simulink model "udp_conn"  (R2016b)
settings: Solver=FixedStepDiscrete  StartTime=0.0  StopTime=5  RelTol=1e-3  EnableMultiTasking=on
undefined symbols (not defined in the file): sldrtexcb_modeswitch, Standard_Devices, UDP_Protocol
libraries: sldrtlib x4, xpcseriallib x1
Description:
  | Packet Input/Output
  | 
  | The example model "sldrtex_packetio" shows how to transfer data through UDP
  | communication protocol using binary encoding. The model sends data
  | within one computer, from one UDP port to another. You can modify the
  | model to communicate between two computers by splitting this model
  | into its send and receive parts and running the models on two computers.
  | The yellow blocks are used to send the data, the blue blocks
  | are used to receive the data. Then, please enter the IP addresses of the two
  | computers into the appropriate fields in the Board Setup dialog.
  | 
  | How to run this model in Normal Mode:
  | 
  | 1) Double-click the orange button to switch to Normal Mode if needed.
  | 2) Start the real-time execution using Simulation->Run.
  | 
  | How to run this model in External Mode:
  | 
  | 1) Double-click the orange button to switch to External Mode if needed.
  | 2) Start the real-time execution using Simulation->Run. The model will automatically
  |    build, connect to Simulink in External Mode and start.
settings Model: SimulationMode=external  ExtModeTrigDuration=1001  Creator=The MathWorks, Inc.  LastModifiedBy=gylaszlo
settings DataIOCC: LimitDataPoints=on  SaveFormat=Array
settings OptimizationCC: ExpressionDepthLimit=2147483647  InitFltsAndDblsToZero=on  EfficientMapNaN2IntZero=off  LifeSpan=inf
settings DebuggingCC: UnderspecifiedInitializationDetection=Classic  MergeDetectMultiDrivingBlocksExec=none  SolverPrmCheckMsg=warning  FcnCallInpInsideContextMsg=warning  AllowSymbolicDim=off  StateNameClashWarn=warning  SFUnexpectedBacktrackingDiag=warning  SFNoUnconditionalDefaultTransitionDiag=warning  SFExecutionAtInitializationDiag=none
settings HardwareCC: TargetBitPerLong=64  TargetBitPerPointer=64  TargetBitPerSizeT=64  TargetBitPerPtrDiffT=64  TargetIntDivRoundTo=Zero  TargetEndianess=LittleEndian  TargetWordSize=64  TargetHWDeviceType=Intel->x86-64
settings ModelReferenceCC: PropagateSignalLabelsOutOfModel=off
settings RTWCC: SystemTargetFile=sldrt.tlc  TemplateMakefile=sldrt.tmf  Description=Simulink Desktop Real-Time  RTWCompilerOptimization=on
settings CodeAppCC: MaxIdLength=95
settings SimulinkDesktopRealTimeCC: TargetPreCompLibLocation=C:\Program Files\MATLAB\R2016b\toolbox\sldrt\lib\win64  TargetLangStandard=C89/C90 (ANSI)  GeneratePreprocessorConditionals=Disable all  SupportVariableSizeSignals=off
settings ConfigComp: CovMetricSettings=dw  CovHtmlReporting=on  CovSaveCumulativeToWorkspaceVar=on  CovSaveSingleToWorkspaceVar=on  CovShowResultsExplorer=off  CovExternalEMLEnable=off  CovSFcnEnable=off

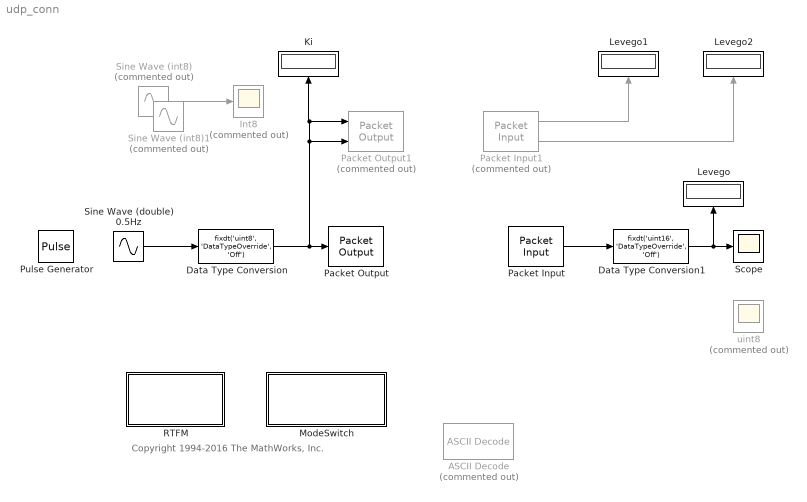
== system udp_conn ==
  note: Copyright 1994-2016 The MathWorks, Inc.
  "ASCII Decode " : xpcseriallib/ASCII Decode   Commented=on  format=%d\r  nvars=1  vartypes={ }
  Data Type Conversion : DataTypeConversion  OutDataTypeStr=fixdt('uint8', 'DataTypeOverride', 'Off')  RndMeth=Nearest  SaturateOnIntegerOverflow=on
  Data Type Conversion1 : DataTypeConversion  OutDataTypeStr=fixdt('uint16', 'DataTypeOverride', 'Off')  RndMeth=Nearest  SaturateOnIntegerOverflow=on  LockScale=on
  Int8 : Scope  Commented=on
  Ki : Display
  Levego : Display
  Levego1 : Display
  Levego2 : Display
  ModeSwitch : Subsystem  InitFcn=sldrtexcb_modeswitch('CheckKernel');  mask(Simulink Desktop Real-Time Example Mode Switch){}
      settings: OpenFcn=sldrtexcb_modeswitch(gcbh);
      mask Display: disp('Switch To\nNormal Mode');
  Packet Input : sldrtlib/Packet Input  SampleTime=2  MaxMissedTicks=50  ShowMissedTicks=off  YieldWhenWaiting=off  DrvName=Standard_Devices/UDP_Protocol  DrvAddress=9089  DrvOptions=[3232235628 9090]  PacketSize=2  DataTypes={'uint16'}  ShowReady=off  ShowError=off  PacketID=1  ByteOrder=2  ShowTimestamp=off
      settings: AttributesFormatString=Standard Devices\nUDP Protocol [2381h]
  Packet Input1 : sldrtlib/Packet Input  Commented=on  SampleTime=0.5  MaxMissedTicks=50  ShowMissedTicks=off  YieldWhenWaiting=off  DrvName=Standard_Devices/UDP_Protocol  DrvAddress=36880  DrvOptions=[2130706433 36864]  PacketSize=2  DataTypes={'uint8', 'int8'}  ShowReady=off  ShowError=off  PacketID=1  ByteOrder=1  ShowTimestamp=off
      settings: AttributesFormatString=Standard Devices\nUDP Protocol [9010h]
  Packet Output : sldrtlib/Packet Output  SampleTime=2  MaxMissedTicks=50  ShowMissedTicks=off  YieldWhenWaiting=off  DrvName=Standard_Devices/UDP_Protocol  DrvAddress=9089  DrvOptions=[3232235628 9090]  PacketSize=1  DataTypes={'uint8'}  ShowReady=off  ShowError=off  PacketID=1  ByteOrder=1  InitialValue=[]  FinalValue=[]
      settings: AttributesFormatString=Standard Devices\nUDP Protocol [2381h]
  Packet Output1 : sldrtlib/Packet Output  Commented=on  SampleTime=0.5  MaxMissedTicks=50  ShowMissedTicks=off  YieldWhenWaiting=off  DrvName=Standard_Devices/UDP_Protocol  DrvAddress=36880  DrvOptions=[2130706433 36864]  PacketSize=2  DataTypes={'uint8', 'int8'}  ShowReady=off  ShowError=off  PacketID=1  ByteOrder=1  InitialValue=[]  FinalValue=[]
      settings: AttributesFormatString=Standard Devices\nUDP Protocol [9010h]
  Pulse Generator : DiscretePulseGenerator  Amplitude=99  Period=10  PulseWidth=5  SampleTime=2
  "RTFM " : Subsystem  mask(Simulink Desktop Real-Time Example Info){}
      settings: OpenFcn=web([docroot '/sldrt/examples/packet-input-output.html']);
      mask Display: disp('Info')
  Scope : Scope
  Sine Wave (double) 0.5Hz : Sin  Amplitude=50  Bias=50  Frequency=0.62*0.5  SampleTime=0
  Sine Wave (int8) : Sin  Commented=on  Amplitude=1:8  Frequency=2  SampleTime=0
  Sine Wave (int8)1 : Sin  Commented=on  Amplitude=1:8  Frequency=2  SampleTime=0
  uint8 : Scope  Commented=on
  wires:
  Data Type Conversion1/1 -> Levego/1, Scope/1
  Sine Wave (int8)/1 -> Int8/1
  Data Type Conversion/1 -> Packet Output/1, Packet Output1/1, Ki/1, Packet Output1/2
  Packet Input/1 -> Data Type Conversion1/1
  Sine Wave (double) 0.5Hz/1 -> Data Type Conversion/1
  Packet Input1/1 -> Levego1/1
  Packet Input1/2 -> Levego2/1

== system udp_conn/ModeSwitch ==

== system udp_conn/RTFM  ==
